simulink model "coefficient_of_lineequation"  (R2022b)
settings: Solver=VariableStepAuto  StartTime=0.0  StopTime=10.0  RelTol=1e-3
settings Model: Creator=XinyiWu  LastModifiedBy=XinyiWu

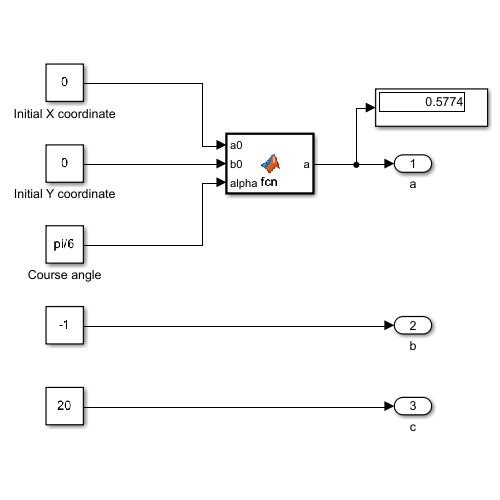
[thumbnail: Simulink's stored preview of the top-level diagram]
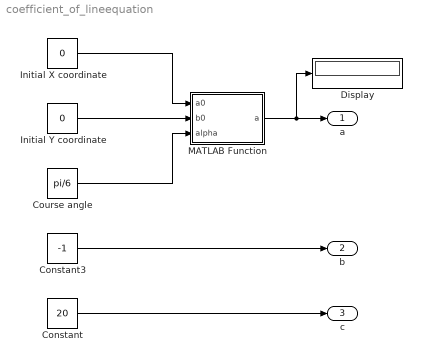
== system coefficient_of_lineequation ==
  Constant : Constant  Value=20
  Constant3 : Constant  Value=-1
  Course angle : Constant  Value=pi/6
  Display : Display
  Initial X coordinate : Constant  Value=0
  Initial Y coordinate : Constant  Value=0
  MATLAB Function : MATLAB Function  TreatAsAtomicUnit=on
  a : Outport
  b : Outport  Port=2
  c : Outport  Port=3
  wires:
  Course angle/1 -> MATLAB Function/3(alpha)
  Initial Y coordinate/1 -> MATLAB Function/2(b0)
  Initial X coordinate/1 -> MATLAB Function/1(a0)
  MATLAB Function/1(a) -> Display/1, a/1
  Constant3/1 -> b/1
  Constant/1 -> c/1

== matlab function coefficient_of_lineequation/MATLAB Function ==
  data: a0 input; a output; b0 input; alpha input
function a = fcn(a0,b0,alpha)

L=515 %meter

if alpha>0
    a = (b0+515*sin(alpha)-b0)/(a0+515*cos(alpha)-a0)
else
    a = (b0-515*sin(alpha)-b0)/(a0+515*cos(alpha)-a0)
end
